simulink model "test_sig_noise"  (Simulink 7.8)
settings: Solver=ode45  StartTime=0.0  StopTime=4e-4  RelTol=1e-3
undefined symbols (not defined in the file): dt_sim, frev_476, Fs_adc
libraries: simulink x3
settings Model: Creator=lucas.russo  LastModifiedBy=lucas.russo

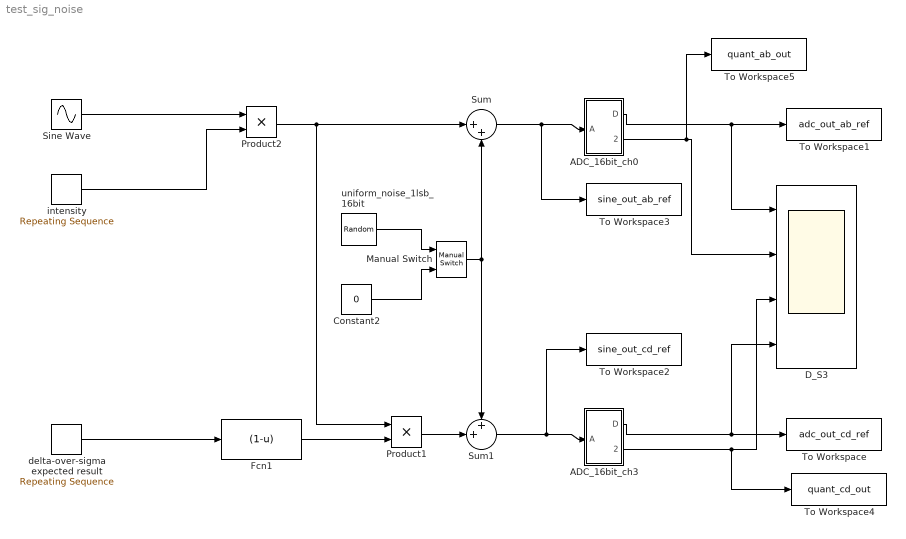
== system test_sig_noise ==
  ADC_16bit_ch0 : Subsystem
  ADC_16bit_ch3 : Subsystem
  Constant2 : Constant  Value=0  SampleTime=0
  D_S3 : Scope  NumInputPorts=4
      settings: TimeRange=0.0004  YMin=-1.5~-1.5~10~-1.5  YMax=1.5~1.5~100~1.5  MaxDataPoints=1000000  SampleInput=on  SampleTime=1e-11
  Fcn1 : Fcn  Expr=(1-u)
  Manual Switch : simulink/Signal Routing/Manual Switch  sw=0  action=0  varsize=off
  Product1 : Product  RndMeth=Zero
  Product2 : Product  RndMeth=Zero
  Sine Wave : Sin  Frequency=2*pi*frev_476  SampleTime=0
  Sum : Sum  Inputs=|++
  Sum1 : Sum  Inputs=++|
  To Workspace : ToWorkspace  VariableName=adc_out_cd_ref  SampleTime=-1  SaveFormat=Structure With Time
  To Workspace1 : ToWorkspace  VariableName=adc_out_ab_ref  SampleTime=-1  SaveFormat=Structure With Time
  To Workspace2 : ToWorkspace  VariableName=sine_out_cd_ref  SampleTime=-1  SaveFormat=Structure With Time
  To Workspace3 : ToWorkspace  VariableName=sine_out_ab_ref  SampleTime=-1  SaveFormat=Structure With Time
  To Workspace4 : ToWorkspace  VariableName=quant_cd_out  SampleTime=-1  SaveFormat=Structure With Time
  To Workspace5 : ToWorkspace  VariableName=quant_ab_out  SampleTime=-1  SaveFormat=Structure With Time
  delta-over-sigma expected result : simulink/Sources/Repeating Sequence  rep_seq_t=[0 0.25e-4 0.25e-4 0.5e-4 0.5e-4 0.75e-4 0.75e-4 1e-4]  rep_seq_y=vrms_att
  intensity : simulink/Sources/Repeating Sequence  rep_seq_t=[0 1e-4 1e-4 2e-4 2e-4 3e-4 3e-4 4e-4]  rep_seq_y=[1 1 0.1 0.1 0.01 0.01 0.001 0.001]
  uniform_noise_1lsb_16bit : UniformRandomNumber  Minimum=-0.5*(2/2^16)  Maximum=0.5*(2/2^16)  Seed=49728613  SampleTime=0
  wires:
  intensity/1 -> Product2/2
  Product2/1 -> Product1/1, Sum/1
  delta-over-sigma expected result/1 -> Fcn1/1
  Fcn1/1 -> Product1/2
  Sine Wave/1 -> Product2/1
  ADC_16bit_ch0/1(D) -> To Workspace1/1, D_S3/1
  ADC_16bit_ch3/1(D) -> D_S3/4, To Workspace/1
  uniform_noise_1lsb_16bit/1 -> Manual Switch/1
  Constant2/1 -> Manual Switch/2
  Sum/1 -> ADC_16bit_ch0/1(A), To Workspace3/1
  Manual Switch/1 -> Sum/2, Sum1/1
  Product1/1 -> Sum1/2
  Sum1/1 -> ADC_16bit_ch3/1(A), To Workspace2/1
  ADC_16bit_ch0/2(Quant) -> D_S3/2, To Workspace5/1
  ADC_16bit_ch3/2(Quant) -> D_S3/3, To Workspace4/1

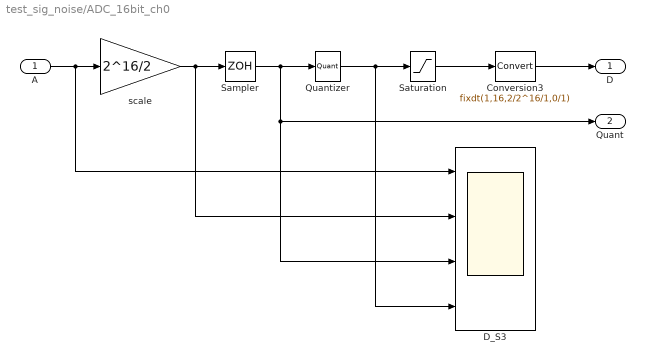
== system test_sig_noise/ADC_16bit_ch0 ==
  A : Inport  OutDataTypeStr=double
  Conversion3 : DataTypeConversion  OutDataTypeStr=fixdt(1,16,2/2^16/1,0/1)  ConvertRealWorld=Stored Integer (SI)  LockScale=on
  D_S3 : Scope  NumInputPorts=4
      settings: TimeRange=0.0004  YMin=-1.5~-1.5~10~-1.5  YMax=1.5~1.5~100~1.5  MaxDataPoints=1000000  SampleInput=on  SampleTime=1e-11
  Quantizer : Quantizer  QuantizationInterval=1  SampleTime=dt_sim
  Sampler : ZeroOrderHold  SampleTime=1/Fs_adc
  Saturation : Saturate  UpperLimit=65536/2-1  LowerLimit=-65536/2  OutDataTypeStr=Inherit: Inherit via back propagation
  scale : Gain  Gain=2^16/2  SaturateOnIntegerOverflow=on  OutDataTypeStr=Inherit: Same as input  ParamDataTypeStr=Inherit: Same as input
  D : Outport
  Quant : Outport  Port=2
  wires:
  A/1 -> scale/1, D_S3/1
  Conversion3/1 -> D/1
  Quantizer/1 -> Saturation/1, D_S3/4
  Sampler/1 -> Quantizer/1, D_S3/3, Quant/1
  Saturation/1 -> Conversion3/1
  scale/1 -> Sampler/1, D_S3/2

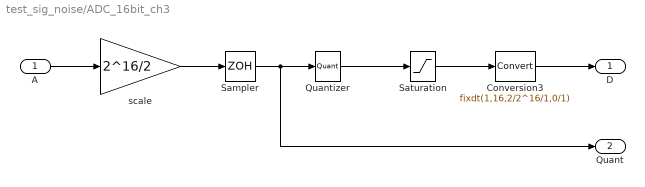
== system test_sig_noise/ADC_16bit_ch3 ==
  A : Inport  OutDataTypeStr=double
  Conversion3 : DataTypeConversion  OutDataTypeStr=fixdt(1,16,2/2^16/1,0/1)  ConvertRealWorld=Stored Integer (SI)  LockScale=on
  Quantizer : Quantizer  QuantizationInterval=1  SampleTime=dt_sim
  Sampler : ZeroOrderHold  SampleTime=1/Fs_adc
  Saturation : Saturate  UpperLimit=65536/2-1  LowerLimit=-65536/2  OutDataTypeStr=Inherit: Inherit via back propagation
  scale : Gain  Gain=2^16/2  SaturateOnIntegerOverflow=on  OutDataTypeStr=Inherit: Same as input  ParamDataTypeStr=Inherit: Same as input
  D : Outport
  Quant : Outport  Port=2
  wires:
  A/1 -> scale/1
  Conversion3/1 -> D/1
  Quantizer/1 -> Saturation/1
  Sampler/1 -> Quantizer/1, Quant/1
  Saturation/1 -> Conversion3/1
  scale/1 -> Sampler/1
